simulink model "TestStructure"  (R2023b)
settings: Solver=FixedStepDiscrete  StartTime=0.0  StopTime=inf  FixedStep=SampleTime  RelTol=1e-3
InitFcn:
  | SampleTime = 0.001;
  | ButtonValue=0;
  | load("BusConfig.mat");
undefined symbols (not defined in the file): DiscIntNeverNeededParam
libraries: slrealtimeethercatlib x219, dspfdesign x28, dspstat3 x23, simulink x21, slpidlib x10, dspswit3 x8, commfilt2 x2, dspsigops x1
(part 5 of 8)

== system TestStructure/Robot/MotorPositonInit1/Subsystem3 ==
  MotorDesirePos : Inport
  MotorPos : Inport  Port=2
  MotorVel : Inport  Port=3
  Discrete PID Controller : slpidlib/PID Controller  Controller=PID  Form=Parallel  TimeDomain=Discrete-time  UseExternalTs=off  SampleTime=-1  IntegratorMethod=Forward Euler  FilterMethod=Forward Euler  ControllerParametersSource=internal  P=220  I=1  UseKiTs=off  D=0.5  N=100  UseFilter=on  TunerSelectOption=Transfer Function Based (PID Tuner App)  InitialConditionSource=internal  InitialConditionForIntegrator=0  InitialConditionForFilter=0  DifferentiatorICPrevScaledInput=0  ExternalReset=none  TrackingMode=off  Kt=1  LimitOutput=off  SatLimitsSource=internal  UpperSaturationLimit=inf  LowerSaturationLimit=-inf  LinearizeAsGain=off  AntiWindupMode=none  Kb=1  LimitIntegrator=off  UpperIntegratorSaturationLimit=inf  LowerIntegratorSaturationLimit=-inf  POutMin=[]  POutMax=[]  IOutMin=[]  IOutMax=[]  DOutMin=[]  DOutMax=[]  NOutMin=[]  NOutMax=[]  SumOutMin=[]  SumOutMax=[]  SaturationOutMin=[]  SaturationOutMax=[]  PParamMin=[]  PParamMax=[]  IParamMin=[]  IParamMax=[]  DParamMin=[]  DParamMax=[]  NParamMin=[]  NParamMax=[]  KbParamMin=[]  KbParamMax=[]  KtParamMin=[]  KtParamMax=[]  KbOutMin=[]  KbOutMax=[]  KtOutMin=[]  KtOutMax=[]  IntegratorOutMin=[]  IntegratorOutMax=[]  FilterOutMin=[]  FilterOutMax=[]  SumI1OutMin=[]  SumI1OutMax=[]  SumI2OutMin=[]  SumI2OutMax=[]  SumI3OutMin=[]  SumI3OutMax=[]  SumI4OutMin=[]  SumI4OutMax=[]  SumDOutMin=[]  SumDOutMax=[]  DifferentiatorOutMin=[]  DifferentiatorOutMax=[]  FilterDiffOutCoefMin=[]  FilterDiffOutCoefMax=[]  ReciprocalOutMin=[]  ReciprocalOutMax=[]  SumDenOutMin=[]  SumDenOutMax=[]  SumNumOutMin=[]  SumNumOutMax=[]  DivideOutMin=[]  DivideOutMax=[]  UdiffTsProdOutMin=[]  UdiffTsProdOutMax=[]  NTsProdOutMin=[]  NTsProdOutMax=[]  UintegralTsProdOutMin=[]  UintegralTsProdOutMax=[]  UngainTsProdOutMin=[]  UngainTsProdOutMax=[]  ClampingZeroOutDataTypeStr=Inherit: Inherit via back propagation  ClampingZeroOutMin=[]  ClampingZeroOutMax=[]  FilterDenConstantOutDataTypeStr=Inherit: Inherit via back propagation  FilterDenConstantOutMin=[]  FilterDenConstantOutMax=[]  PCopyOutDataTypeStr=Inherit: Inherit via back propagation  PCopyOutMin=[]  PCopyOutMax=[]  NCopyOutDataTypeStr=Inherit: Inherit via back propagation  NCopyOutMin=[]  NCopyOutMax=[]  IntegratorContinuousStateAttributes=''  IntegratorStateMustResolveToSignalObject=off  IntegratorRTWStateStorageClass=Auto  FilterContinuousStateAttributes=''  FilterStateMustResolveToSignalObject=off  FilterRTWStateStorageClass=Auto  ParallelPVariant=InternalParameters  IdealPVariant=Disabled  IVariant=InternalParameters  DVariant=InternalParameters  IntegratorVariant=Discrete  SatVariant=Disabled  AWVariant=Passthrough  PCopyVariant=Disabled  TRVariant=Disabled  FdbkBlocksVariant=Forward  IdealPFdbkVariant=Disabled  SatFdbkVariant=Disabled  DerivativeFilterVariant=ForwardEulerFilter  NVariant=InternalParameters  NCopyVariant=Disabled  FilterICVariant=InternalICsFilter  IntegratorICVariant=InternalICs  ExternalResetVariant=Disabled  TRSumVariant=Passthrough  SumFdbkVariant=Disabled  SumVariant=Sum_PID  TsampFilterVariant=InternalTs  TsampNgainVariant=Passthrough  TsampIntegralVariant=Disabled_SignalSpec  ExternalSaturationOutDataTypeStr=Inherit: Same as second input
      settings: LibrarySourceBlock=simulink/Discrete/Discrete PID Controller
  Discrete PID Controller1 : slpidlib/PID Controller  Controller=PD  Form=Parallel  TimeDomain=Discrete-time  UseExternalTs=off  SampleTime=-1  IntegratorMethod=Forward Euler  FilterMethod=Forward Euler  ControllerParametersSource=internal  P=0.0035  I=1  UseKiTs=off  D=0.00005  N=100  UseFilter=on  TunerSelectOption=Transfer Function Based (PID Tuner App)  InitialConditionSource=internal  InitialConditionForIntegrator=0  InitialConditionForFilter=0  DifferentiatorICPrevScaledInput=0  ExternalReset=none  TrackingMode=off  Kt=1  LimitOutput=on  SatLimitsSource=internal  UpperSaturationLimit=15  LowerSaturationLimit=-15  LinearizeAsGain=off  AntiWindupMode=none  Kb=1  LimitIntegrator=off  UpperIntegratorSaturationLimit=inf  LowerIntegratorSaturationLimit=-inf  POutMin=[]  POutMax=[]  IOutMin=[]  IOutMax=[]  DOutMin=[]  DOutMax=[]  NOutMin=[]  NOutMax=[]  SumOutMin=[]  SumOutMax=[]  SaturationOutMin=[]  SaturationOutMax=[]  PParamMin=[]  PParamMax=[]  IParamMin=[]  IParamMax=[]  DParamMin=[]  DParamMax=[]  NParamMin=[]  NParamMax=[]  KbParamMin=[]  KbParamMax=[]  KtParamMin=[]  KtParamMax=[]  KbOutMin=[]  KbOutMax=[]  KtOutMin=[]  KtOutMax=[]  IntegratorOutMin=[]  IntegratorOutMax=[]  FilterOutMin=[]  FilterOutMax=[]  SumI1OutMin=[]  SumI1OutMax=[]  SumI2OutMin=[]  SumI2OutMax=[]  SumI3OutMin=[]  SumI3OutMax=[]  SumI4OutMin=[]  SumI4OutMax=[]  SumDOutMin=[]  SumDOutMax=[]  DifferentiatorOutMin=[]  DifferentiatorOutMax=[]  FilterDiffOutCoefMin=[]  FilterDiffOutCoefMax=[]  ReciprocalOutMin=[]  ReciprocalOutMax=[]  SumDenOutMin=[]  SumDenOutMax=[]  SumNumOutMin=[]  SumNumOutMax=[]  DivideOutMin=[]  DivideOutMax=[]  UdiffTsProdOutMin=[]  UdiffTsProdOutMax=[]  NTsProdOutMin=[]  NTsProdOutMax=[]  UintegralTsProdOutMin=[]  UintegralTsProdOutMax=[]  UngainTsProdOutMin=[]  UngainTsProdOutMax=[]  ClampingZeroOutDataTypeStr=Inherit: Inherit via back propagation  ClampingZeroOutMin=[]  ClampingZeroOutMax=[]  FilterDenConstantOutDataTypeStr=Inherit: Inherit via back propagation  FilterDenConstantOutMin=[]  FilterDenConstantOutMax=[]  PCopyOutDataTypeStr=Inherit: Inherit via back propagation  PCopyOutMin=[]  PCopyOutMax=[]  NCopyOutDataTypeStr=Inherit: Inherit via back propagation  NCopyOutMin=[]  NCopyOutMax=[]  IntegratorContinuousStateAttributes=''  IntegratorStateMustResolveToSignalObject=off  IntegratorRTWStateStorageClass=Auto  FilterContinuousStateAttributes=''  FilterStateMustResolveToSignalObject=off  FilterRTWStateStorageClass=Auto  ParallelPVariant=InternalParameters  IdealPVariant=Disabled  IVariant=Disabled  DVariant=InternalParameters  IntegratorVariant=Disabled  SatVariant=Enabled  AWVariant=Disabled  PCopyVariant=Disabled  TRVariant=Disabled  FdbkBlocksVariant=Forward  IdealPFdbkVariant=Disabled  SatFdbkVariant=Disabled  DerivativeFilterVariant=ForwardEulerFilter  NVariant=InternalParameters  NCopyVariant=Disabled  FilterICVariant=InternalICsFilter  IntegratorICVariant=Disabled  ExternalResetVariant=Disabled  TRSumVariant=Passthrough  SumFdbkVariant=Disabled  SumVariant=Sum_PD  TsampFilterVariant=InternalTs  TsampNgainVariant=Passthrough  TsampIntegralVariant=Disabled_SignalSpec  ExternalSaturationOutDataTypeStr=Inherit: Same as second input
      settings: LibrarySourceBlock=simulink/Discrete/Discrete PID Controller
  Saturation1 : Saturate  UpperLimit=60  LowerLimit=-60
  Sum : Sum  Inputs=|+-
  Sum1 : Sum  Inputs=|+-
  MotorTorque : Outport
  wires:
  Discrete PID Controller1/1 -> MotorTorque/1
  Sum/1 -> Discrete PID Controller/1
  Saturation1/1 -> Sum1/2
  Discrete PID Controller/1 -> Sum1/1
  Sum1/1 -> Discrete PID Controller1/1
  MotorDesirePos/1 -> Sum/1
  MotorVel/1 -> Saturation1/1
  MotorPos/1 -> Sum/2

== system TestStructure/Robot/MotorPositonInit1/Subsystem4 ==
  MotorDesirePos : Inport
  MotorPos : Inport  Port=2
  MotorVel : Inport  Port=3
  Discrete PID Controller : slpidlib/PID Controller  Controller=PID  Form=Parallel  TimeDomain=Discrete-time  UseExternalTs=off  SampleTime=-1  IntegratorMethod=Forward Euler  FilterMethod=Forward Euler  ControllerParametersSource=internal  P=220  I=1  UseKiTs=off  D=2  N=100  UseFilter=on  TunerSelectOption=Transfer Function Based (PID Tuner App)  InitialConditionSource=internal  InitialConditionForIntegrator=0  InitialConditionForFilter=0  DifferentiatorICPrevScaledInput=0  ExternalReset=none  TrackingMode=off  Kt=1  LimitOutput=off  SatLimitsSource=internal  UpperSaturationLimit=inf  LowerSaturationLimit=-inf  LinearizeAsGain=off  AntiWindupMode=none  Kb=1  LimitIntegrator=off  UpperIntegratorSaturationLimit=inf  LowerIntegratorSaturationLimit=-inf  POutMin=[]  POutMax=[]  IOutMin=[]  IOutMax=[]  DOutMin=[]  DOutMax=[]  NOutMin=[]  NOutMax=[]  SumOutMin=[]  SumOutMax=[]  SaturationOutMin=[]  SaturationOutMax=[]  PParamMin=[]  PParamMax=[]  IParamMin=[]  IParamMax=[]  DParamMin=[]  DParamMax=[]  NParamMin=[]  NParamMax=[]  KbParamMin=[]  KbParamMax=[]  KtParamMin=[]  KtParamMax=[]  KbOutMin=[]  KbOutMax=[]  KtOutMin=[]  KtOutMax=[]  IntegratorOutMin=[]  IntegratorOutMax=[]  FilterOutMin=[]  FilterOutMax=[]  SumI1OutMin=[]  SumI1OutMax=[]  SumI2OutMin=[]  SumI2OutMax=[]  SumI3OutMin=[]  SumI3OutMax=[]  SumI4OutMin=[]  SumI4OutMax=[]  SumDOutMin=[]  SumDOutMax=[]  DifferentiatorOutMin=[]  DifferentiatorOutMax=[]  FilterDiffOutCoefMin=[]  FilterDiffOutCoefMax=[]  ReciprocalOutMin=[]  ReciprocalOutMax=[]  SumDenOutMin=[]  SumDenOutMax=[]  SumNumOutMin=[]  SumNumOutMax=[]  DivideOutMin=[]  DivideOutMax=[]  UdiffTsProdOutMin=[]  UdiffTsProdOutMax=[]  NTsProdOutMin=[]  NTsProdOutMax=[]  UintegralTsProdOutMin=[]  UintegralTsProdOutMax=[]  UngainTsProdOutMin=[]  UngainTsProdOutMax=[]  ClampingZeroOutDataTypeStr=Inherit: Inherit via back propagation  ClampingZeroOutMin=[]  ClampingZeroOutMax=[]  FilterDenConstantOutDataTypeStr=Inherit: Inherit via back propagation  FilterDenConstantOutMin=[]  FilterDenConstantOutMax=[]  PCopyOutDataTypeStr=Inherit: Inherit via back propagation  PCopyOutMin=[]  PCopyOutMax=[]  NCopyOutDataTypeStr=Inherit: Inherit via back propagation  NCopyOutMin=[]  NCopyOutMax=[]  IntegratorContinuousStateAttributes=''  IntegratorStateMustResolveToSignalObject=off  IntegratorRTWStateStorageClass=Auto  FilterContinuousStateAttributes=''  FilterStateMustResolveToSignalObject=off  FilterRTWStateStorageClass=Auto  ParallelPVariant=InternalParameters  IdealPVariant=Disabled  IVariant=InternalParameters  DVariant=InternalParameters  IntegratorVariant=Discrete  SatVariant=Disabled  AWVariant=Passthrough  PCopyVariant=Disabled  TRVariant=Disabled  FdbkBlocksVariant=Forward  IdealPFdbkVariant=Disabled  SatFdbkVariant=Disabled  DerivativeFilterVariant=ForwardEulerFilter  NVariant=InternalParameters  NCopyVariant=Disabled  FilterICVariant=InternalICsFilter  IntegratorICVariant=InternalICs  ExternalResetVariant=Disabled  TRSumVariant=Passthrough  SumFdbkVariant=Disabled  SumVariant=Sum_PID  TsampFilterVariant=InternalTs  TsampNgainVariant=Passthrough  TsampIntegralVariant=Disabled_SignalSpec  ExternalSaturationOutDataTypeStr=Inherit: Same as second input
      settings: LibrarySourceBlock=simulink/Discrete/Discrete PID Controller
  Discrete PID Controller1 : slpidlib/PID Controller  Controller=PD  Form=Parallel  TimeDomain=Discrete-time  UseExternalTs=off  SampleTime=-1  IntegratorMethod=Forward Euler  FilterMethod=Forward Euler  ControllerParametersSource=internal  P=0.0035  I=1  UseKiTs=off  D=0.00005  N=100  UseFilter=on  TunerSelectOption=Transfer Function Based (PID Tuner App)  InitialConditionSource=internal  InitialConditionForIntegrator=0  InitialConditionForFilter=0  DifferentiatorICPrevScaledInput=0  ExternalReset=none  TrackingMode=off  Kt=1  LimitOutput=on  SatLimitsSource=internal  UpperSaturationLimit=15  LowerSaturationLimit=-15  LinearizeAsGain=off  AntiWindupMode=none  Kb=1  LimitIntegrator=off  UpperIntegratorSaturationLimit=inf  LowerIntegratorSaturationLimit=-inf  POutMin=[]  POutMax=[]  IOutMin=[]  IOutMax=[]  DOutMin=[]  DOutMax=[]  NOutMin=[]  NOutMax=[]  SumOutMin=[]  SumOutMax=[]  SaturationOutMin=[]  SaturationOutMax=[]  PParamMin=[]  PParamMax=[]  IParamMin=[]  IParamMax=[]  DParamMin=[]  DParamMax=[]  NParamMin=[]  NParamMax=[]  KbParamMin=[]  KbParamMax=[]  KtParamMin=[]  KtParamMax=[]  KbOutMin=[]  KbOutMax=[]  KtOutMin=[]  KtOutMax=[]  IntegratorOutMin=[]  IntegratorOutMax=[]  FilterOutMin=[]  FilterOutMax=[]  SumI1OutMin=[]  SumI1OutMax=[]  SumI2OutMin=[]  SumI2OutMax=[]  SumI3OutMin=[]  SumI3OutMax=[]  SumI4OutMin=[]  SumI4OutMax=[]  SumDOutMin=[]  SumDOutMax=[]  DifferentiatorOutMin=[]  DifferentiatorOutMax=[]  FilterDiffOutCoefMin=[]  FilterDiffOutCoefMax=[]  ReciprocalOutMin=[]  ReciprocalOutMax=[]  SumDenOutMin=[]  SumDenOutMax=[]  SumNumOutMin=[]  SumNumOutMax=[]  DivideOutMin=[]  DivideOutMax=[]  UdiffTsProdOutMin=[]  UdiffTsProdOutMax=[]  NTsProdOutMin=[]  NTsProdOutMax=[]  UintegralTsProdOutMin=[]  UintegralTsProdOutMax=[]  UngainTsProdOutMin=[]  UngainTsProdOutMax=[]  ClampingZeroOutDataTypeStr=Inherit: Inherit via back propagation  ClampingZeroOutMin=[]  ClampingZeroOutMax=[]  FilterDenConstantOutDataTypeStr=Inherit: Inherit via back propagation  FilterDenConstantOutMin=[]  FilterDenConstantOutMax=[]  PCopyOutDataTypeStr=Inherit: Inherit via back propagation  PCopyOutMin=[]  PCopyOutMax=[]  NCopyOutDataTypeStr=Inherit: Inherit via back propagation  NCopyOutMin=[]  NCopyOutMax=[]  IntegratorContinuousStateAttributes=''  IntegratorStateMustResolveToSignalObject=off  IntegratorRTWStateStorageClass=Auto  FilterContinuousStateAttributes=''  FilterStateMustResolveToSignalObject=off  FilterRTWStateStorageClass=Auto  ParallelPVariant=InternalParameters  IdealPVariant=Disabled  IVariant=Disabled  DVariant=InternalParameters  IntegratorVariant=Disabled  SatVariant=Enabled  AWVariant=Disabled  PCopyVariant=Disabled  TRVariant=Disabled  FdbkBlocksVariant=Forward  IdealPFdbkVariant=Disabled  SatFdbkVariant=Disabled  DerivativeFilterVariant=ForwardEulerFilter  NVariant=InternalParameters  NCopyVariant=Disabled  FilterICVariant=InternalICsFilter  IntegratorICVariant=Disabled  ExternalResetVariant=Disabled  TRSumVariant=Passthrough  SumFdbkVariant=Disabled  SumVariant=Sum_PD  TsampFilterVariant=InternalTs  TsampNgainVariant=Passthrough  TsampIntegralVariant=Disabled_SignalSpec  ExternalSaturationOutDataTypeStr=Inherit: Same as second input
      settings: LibrarySourceBlock=simulink/Discrete/Discrete PID Controller
  Saturation1 : Saturate  UpperLimit=60  LowerLimit=-60
  Sum : Sum  Inputs=|+-
  Sum1 : Sum  Inputs=|+-
  MotorTorque : Outport
  wires:
  Discrete PID Controller1/1 -> MotorTorque/1
  Sum/1 -> Discrete PID Controller/1
  Saturation1/1 -> Sum1/2
  Discrete PID Controller/1 -> Sum1/1
  Sum1/1 -> Discrete PID Controller1/1
  MotorDesirePos/1 -> Sum/1
  MotorVel/1 -> Saturation1/1
  MotorPos/1 -> Sum/2

== system TestStructure/Bus/Subsystem6/Enabled Subsystem/Subsystem ==
  In1 : Inport
  In2 : Inport  Port=2
  In3 : Inport  Port=3
  In4 : Inport  Port=4
  EtherCAT PDO Receive1 : slrealtimeethercatlib/EtherCAT PDO Receive  Priority=2  sig_name=Box 1 (PIC32 EtherCAT Slave01).INPUTS process data mapping.FORCE1  sig_offset=696  sig_type=single  type_size=32  sig_dim=1  device_id=0  sample_time=0.001
  EtherCAT PDO Receive2 : slrealtimeethercatlib/EtherCAT PDO Receive  Priority=2  sig_name=Box 1 (PIC32 EtherCAT Slave01).INPUTS process data mapping.FORCE2  sig_offset=728  sig_type=single  type_size=32  sig_dim=1  device_id=0  sample_time=0.001000
  EtherCAT PDO Receive3 : slrealtimeethercatlib/EtherCAT PDO Receive  Priority=2  sig_name=Box 1 (PIC32 EtherCAT Slave01).INPUTS process data mapping.IMU1_X  sig_offset=952  sig_type=single  type_size=32  sig_dim=1  device_id=0  sample_time=0.001000
  EtherCAT PDO Receive4 : slrealtimeethercatlib/EtherCAT PDO Receive  Priority=2  sig_name=Box 1 (PIC32 EtherCAT Slave01).INPUTS process data mapping.IMU1_Y  sig_offset=984  sig_type=single  type_size=32  sig_dim=1  device_id=0  sample_time=0.001000
  EtherCAT PDO Receive5 : slrealtimeethercatlib/EtherCAT PDO Receive  Priority=2  sig_name=Box 1 (PIC32 EtherCAT Slave01).INPUTS process data mapping.IMU1_Z  sig_offset=1016  sig_type=single  type_size=32  sig_dim=1  device_id=0  sample_time=0.001000
  EtherCAT PDO Receive6 : slrealtimeethercatlib/EtherCAT PDO Receive  Priority=2  sig_name=Box 1 (PIC32 EtherCAT Slave01).INPUTS process data mapping.IMU2_X  sig_offset=1048  sig_type=single  type_size=32  sig_dim=1  device_id=0  sample_time=0.001000
  EtherCAT PDO Receive7 : slrealtimeethercatlib/EtherCAT PDO Receive  Priority=2  sig_name=Box 1 (PIC32 EtherCAT Slave01).INPUTS process data mapping.FORCE3  sig_offset=760  sig_type=single  type_size=32  sig_dim=1  device_id=0  sample_time=0.001000
  EtherCAT PDO Receive8 : slrealtimeethercatlib/EtherCAT PDO Receive  Priority=2  sig_name=Box 1 (PIC32 EtherCAT Slave01).INPUTS process data mapping.FORCE3  sig_offset=760  sig_type=single  type_size=32  sig_dim=1  device_id=0  sample_time=0.001000
  EtherCAT PDO Receive9 : slrealtimeethercatlib/EtherCAT PDO Receive  Priority=2  sig_name=Box 1 (PIC32 EtherCAT Slave01).INPUTS process data mapping.FORCE3  sig_offset=760  sig_type=single  type_size=32  sig_dim=1  device_id=0  sample_time=0.001000
  EtherCAT PDO Transmit{,1..3} (4 alike) : slrealtimeethercatlib/EtherCAT PDO Transmit  Priority=5  sig_name=Drive 2 (Elmo Drive ).Outputs.Target Torque  sig_offset=12496  sig_type=int16  type_size=16  sig_dim=1  device_id=0  sample_time=0.001000
  Out1 : Outport
  Out2 : Outport  Port=2
  Out3 : Outport  Port=3
  Out4 : Outport  Port=4
  Out5 : Outport  Port=5
  Out6 : Outport  Port=6
  Out7 : Outport  Port=7
  Out8 : Outport  Port=8
  Out9 : Outport  Port=9
  wires:
  EtherCAT PDO Receive1/1 -> Out1/1
  EtherCAT PDO Receive2/1 -> Out2/1
  EtherCAT PDO Receive3/1 -> Out3/1
  EtherCAT PDO Receive4/1 -> Out4/1
  EtherCAT PDO Receive5/1 -> Out5/1
  EtherCAT PDO Receive6/1 -> Out6/1
  EtherCAT PDO Receive7/1 -> Out7/1
  EtherCAT PDO Receive8/1 -> Out8/1
  EtherCAT PDO Receive9/1 -> Out9/1
  In1/1 -> EtherCAT PDO Transmit/1
  In2/1 -> EtherCAT PDO Transmit1/1
  In4/1 -> EtherCAT PDO Transmit2/1
  In3/1 -> EtherCAT PDO Transmit3/1

== system TestStructure/Bus/Subsystem6/Enabled Subsystem/Subsystem1 ==
  In1 : Inport
  EtherCAT PDO Receive1 : slrealtimeethercatlib/EtherCAT PDO Receive  Priority=2  Commented=on  sig_name=Drive 2 (Elmo Drive ).Inputs.Position actual value  sig_offset=12496  sig_type=int32  type_size=32  sig_dim=1  device_id=0  sample_time=0.001000
  EtherCAT PDO Receive2 : slrealtimeethercatlib/EtherCAT PDO Receive  Priority=2  Commented=on  sig_name=Drive 2 (Elmo Drive ).Inputs_1.Velocity actual value  sig_offset=12576  sig_type=int32  type_size=32  sig_dim=1  device_id=0  sample_time=0.001000
  EtherCAT PDO Receive3 : slrealtimeethercatlib/EtherCAT PDO Receive  Priority=2  Commented=on  sig_name=Drive 2 (Elmo Drive ).Inputs.Torque actual value  sig_offset=12528  sig_type=int16  type_size=16  sig_dim=1  device_id=0  sample_time=0.001000
  EtherCAT PDO Receive4 : slrealtimeethercatlib/EtherCAT PDO Receive  Priority=2  Commented=on  sig_name=Drive 2 (Elmo Drive ).Inputs_2.DC link circuit voltage  sig_offset=12608  sig_type=uint32  type_size=32  sig_dim=1  device_id=0  sample_time=0.001000
  EtherCAT PDO Receive5 : slrealtimeethercatlib/EtherCAT PDO Receive  Priority=2  Commented=on  sig_name=Drive 2 (Elmo Drive ).Inputs.Mode of operation display  sig_offset=12560  sig_type=int8  type_size=8  sig_dim=1  device_id=0  sample_time=0.001000
  EtherCAT PDO Transmit : slrealtimeethercatlib/EtherCAT PDO Transmit  Priority=5  sig_name=Drive 3 (Elmo Drive ).Outputs.Target Torque  sig_offset=1432  sig_type=int16  type_size=16  sig_dim=1  device_id=0  sample_time=0.001000
  Out1 : Outport
  Out2 : Outport  Port=2
  Out3 : Outport  Port=3
  Out4 : Outport  Port=4
  Out5 : Outport  Port=5
  wires:
  In1/1 -> EtherCAT PDO Transmit/1
  EtherCAT PDO Receive5/1 -> Out5/1
  EtherCAT PDO Receive4/1 -> Out4/1
  EtherCAT PDO Receive3/1 -> Out3/1
  EtherCAT PDO Receive2/1 -> Out2/1
  EtherCAT PDO Receive1/1 -> Out1/1

== system TestStructure/Bus/Subsystem6/Enabled Subsystem/Subsystem10 ==
  EtherCAT PDO Receive1 : slrealtimeethercatlib/EtherCAT PDO Receive  Priority=2  sig_name=Box 1 (PIC32 EtherCAT Slave01).INPUTS process data mapping.FORCE1  sig_offset=696  sig_type=single  type_size=32  sig_dim=1  device_id=0  sample_time=0.001000
  EtherCAT PDO Receive2 : slrealtimeethercatlib/EtherCAT PDO Receive  Priority=2  sig_name=Box 1 (PIC32 EtherCAT Slave01).INPUTS process data mapping.FORCE2  sig_offset=728  sig_type=single  type_size=32  sig_dim=1  device_id=0  sample_time=0.001000
  EtherCAT PDO Receive3 : slrealtimeethercatlib/EtherCAT PDO Receive  Priority=2  sig_name=Box 1 (PIC32 EtherCAT Slave01).INPUTS process data mapping.IMU1_X  sig_offset=952  sig_type=single  type_size=32  sig_dim=1  device_id=0  sample_time=0.001000
  EtherCAT PDO Receive4 : slrealtimeethercatlib/EtherCAT PDO Receive  Priority=2  sig_name=Box 1 (PIC32 EtherCAT Slave01).INPUTS process data mapping.IMU1_Y  sig_offset=984  sig_type=single  type_size=32  sig_dim=1  device_id=0  sample_time=0.001000
  EtherCAT PDO Receive5 : slrealtimeethercatlib/EtherCAT PDO Receive  Priority=2  sig_name=Box 1 (PIC32 EtherCAT Slave01).INPUTS process data mapping.IMU1_Z  sig_offset=1016  sig_type=single  type_size=32  sig_dim=1  device_id=0  sample_time=0.001000
  EtherCAT PDO Receive6 : slrealtimeethercatlib/EtherCAT PDO Receive  Priority=2  sig_name=Box 1 (PIC32 EtherCAT Slave01).INPUTS process data mapping.IMU2_X  sig_offset=1048  sig_type=single  type_size=32  sig_dim=1  device_id=0  sample_time=0.001000
  EtherCAT PDO Receive7 : slrealtimeethercatlib/EtherCAT PDO Receive  Priority=2  sig_name=Box 1 (PIC32 EtherCAT Slave01).INPUTS process data mapping.FORCE3  sig_offset=760  sig_type=single  type_size=32  sig_dim=1  device_id=0  sample_time=0.001000
  Out1 : Outport
  Out2 : Outport  Port=2
  Out3 : Outport  Port=3
  Out4 : Outport  Port=4
  Out5 : Outport  Port=5
  Out6 : Outport  Port=6
  Out7 : Outport  Port=7
  wires:
  EtherCAT PDO Receive1/1 -> Out1/1
  EtherCAT PDO Receive2/1 -> Out2/1
  EtherCAT PDO Receive3/1 -> Out3/1
  EtherCAT PDO Receive4/1 -> Out4/1
  EtherCAT PDO Receive5/1 -> Out5/1
  EtherCAT PDO Receive6/1 -> Out6/1
  EtherCAT PDO Receive7/1 -> Out7/1

== system TestStructure/Bus/Subsystem6/Enabled Subsystem/Subsystem11 ==
  EtherCAT PDO Receive1 : slrealtimeethercatlib/EtherCAT PDO Receive  Priority=2  sig_name=Box 1 (PIC32 EtherCAT Slave01).INPUTS process data mapping.FORCE1  sig_offset=696  sig_type=single  type_size=32  sig_dim=1  device_id=0  sample_time=0.001000
  EtherCAT PDO Receive2 : slrealtimeethercatlib/EtherCAT PDO Receive  Priority=2  sig_name=Box 1 (PIC32 EtherCAT Slave01).INPUTS process data mapping.FORCE2  sig_offset=728  sig_type=single  type_size=32  sig_dim=1  device_id=0  sample_time=0.001000
  EtherCAT PDO Receive3 : slrealtimeethercatlib/EtherCAT PDO Receive  Priority=2  sig_name=Box 1 (PIC32 EtherCAT Slave01).INPUTS process data mapping.IMU1_X  sig_offset=952  sig_type=single  type_size=32  sig_dim=1  device_id=0  sample_time=0.001000
  EtherCAT PDO Receive4 : slrealtimeethercatlib/EtherCAT PDO Receive  Priority=2  sig_name=Box 1 (PIC32 EtherCAT Slave01).INPUTS process data mapping.IMU1_Y  sig_offset=984  sig_type=single  type_size=32  sig_dim=1  device_id=0  sample_time=0.001000
  EtherCAT PDO Receive5 : slrealtimeethercatlib/EtherCAT PDO Receive  Priority=2  sig_name=Box 1 (PIC32 EtherCAT Slave01).INPUTS process data mapping.IMU1_Z  sig_offset=1016  sig_type=single  type_size=32  sig_dim=1  device_id=0  sample_time=0.001000
  EtherCAT PDO Receive6 : slrealtimeethercatlib/EtherCAT PDO Receive  Priority=2  sig_name=Box 1 (PIC32 EtherCAT Slave01).INPUTS process data mapping.IMU2_X  sig_offset=1048  sig_type=single  type_size=32  sig_dim=1  device_id=0  sample_time=0.001000
  EtherCAT PDO Receive7 : slrealtimeethercatlib/EtherCAT PDO Receive  Priority=2  sig_name=Box 1 (PIC32 EtherCAT Slave01).INPUTS process data mapping.FORCE3  sig_offset=760  sig_type=single  type_size=32  sig_dim=1  device_id=0  sample_time=0.001000
  Out1 : Outport
  Out2 : Outport  Port=2
  Out3 : Outport  Port=3
  Out4 : Outport  Port=4
  Out5 : Outport  Port=5
  Out6 : Outport  Port=6
  Out7 : Outport  Port=7
  wires:
  EtherCAT PDO Receive1/1 -> Out1/1
  EtherCAT PDO Receive2/1 -> Out2/1
  EtherCAT PDO Receive3/1 -> Out3/1
  EtherCAT PDO Receive4/1 -> Out4/1
  EtherCAT PDO Receive5/1 -> Out5/1
  EtherCAT PDO Receive6/1 -> Out6/1
  EtherCAT PDO Receive7/1 -> Out7/1

== system TestStructure/Bus/Subsystem6/Enabled Subsystem/Subsystem2 ==
  In1 : Inport
  EtherCAT PDO Receive1 : slrealtimeethercatlib/EtherCAT PDO Receive  Priority=2  Commented=on  sig_name=Drive 4 (Elmo Drive ).Inputs.Position actual value  sig_offset=37072  sig_type=int32  type_size=32  sig_dim=1  device_id=0  sample_time=0.001000
  EtherCAT PDO Receive2 : slrealtimeethercatlib/EtherCAT PDO Receive  Priority=2  Commented=on  sig_name=Drive 4 (Elmo Drive ).Inputs_1.Velocity actual value  sig_offset=37152  sig_type=int32  type_size=32  sig_dim=1  device_id=0  sample_time=0.001000
  EtherCAT PDO Receive3 : slrealtimeethercatlib/EtherCAT PDO Receive  Priority=2  Commented=on  sig_name=Drive 4 (Elmo Drive ).Inputs.Torque actual value  sig_offset=37104  sig_type=int16  type_size=16  sig_dim=1  device_id=0  sample_time=0.001000
  EtherCAT PDO Receive4 : slrealtimeethercatlib/EtherCAT PDO Receive  Priority=2  Commented=on  sig_name=Drive 4 (Elmo Drive ).Inputs_2.DC link circuit voltage  sig_offset=37184  sig_type=uint32  type_size=32  sig_dim=1  device_id=0  sample_time=0.001000
  EtherCAT PDO Receive5 : slrealtimeethercatlib/EtherCAT PDO Receive  Priority=2  Commented=on  sig_name=Drive 4 (Elmo Drive ).Inputs.Mode of operation display  sig_offset=37136  sig_type=int8  type_size=8  sig_dim=1  device_id=0  sample_time=0.001000
  EtherCAT PDO Transmit : slrealtimeethercatlib/EtherCAT PDO Transmit  Priority=5  sig_name=Drive 6 (Elmo Drive ).Outputs.Target Torque  sig_offset=13232  sig_type=int16  type_size=16  sig_dim=1  device_id=0  sample_time=0.001000
  Out1 : Outport
  Out2 : Outport  Port=2
  Out3 : Outport  Port=3
  Out4 : Outport  Port=4
  Out5 : Outport  Port=5
  wires:
  In1/1 -> EtherCAT PDO Transmit/1
  EtherCAT PDO Receive5/1 -> Out5/1
  EtherCAT PDO Receive4/1 -> Out4/1
  EtherCAT PDO Receive3/1 -> Out3/1
  EtherCAT PDO Receive2/1 -> Out2/1
  EtherCAT PDO Receive1/1 -> Out1/1

== system TestStructure/Bus/Subsystem6/Enabled Subsystem/Subsystem3 ==
  In1 : Inport
  EtherCAT PDO Receive1 : slrealtimeethercatlib/EtherCAT PDO Receive  Priority=2  sig_name=Drive 2 (Elmo Drive ).Inputs.Position actual value  sig_offset=12496  sig_type=int32  type_size=32  sig_dim=1  device_id=0  sample_time=0.001000
  EtherCAT PDO Receive2 : slrealtimeethercatlib/EtherCAT PDO Receive  Priority=2  sig_name=Drive 2 (Elmo Drive ).Inputs_1.Velocity actual value  sig_offset=12576  sig_type=int32  type_size=32  sig_dim=1  device_id=0  sample_time=0.001000
  EtherCAT PDO Receive3 : slrealtimeethercatlib/EtherCAT PDO Receive  Priority=2  sig_name=Drive 2 (Elmo Drive ).Inputs.Torque actual value  sig_offset=12528  sig_type=int16  type_size=16  sig_dim=1  device_id=0  sample_time=0.001000
  EtherCAT PDO Receive4 : slrealtimeethercatlib/EtherCAT PDO Receive  Priority=2  sig_name=Drive 2 (Elmo Drive ).Inputs_2.DC link circuit voltage  sig_offset=12608  sig_type=uint32  type_size=32  sig_dim=1  device_id=0  sample_time=0.001000
  EtherCAT PDO Receive5 : slrealtimeethercatlib/EtherCAT PDO Receive  Priority=2  sig_name=Drive 2 (Elmo Drive ).Inputs.Mode of operation display  sig_offset=12560  sig_type=int8  type_size=8  sig_dim=1  device_id=0  sample_time=0.001000
  EtherCAT PDO Transmit : slrealtimeethercatlib/EtherCAT PDO Transmit  Priority=5  sig_name=Drive 2 (Elmo Drive ).Outputs.Target Torque  sig_offset=12496  sig_type=int16  type_size=16  sig_dim=1  device_id=0  sample_time=0.001000
  Out1 : Outport
  Out2 : Outport  Port=2
  Out3 : Outport  Port=3
  Out4 : Outport  Port=4
  Out5 : Outport  Port=5
  wires:
  In1/1 -> EtherCAT PDO Transmit/1
  EtherCAT PDO Receive5/1 -> Out5/1
  EtherCAT PDO Receive4/1 -> Out4/1
  EtherCAT PDO Receive3/1 -> Out3/1
  EtherCAT PDO Receive2/1 -> Out2/1
  EtherCAT PDO Receive1/1 -> Out1/1

== system TestStructure/Bus/Subsystem6/Enabled Subsystem/Subsystem4 ==
  In1 : Inport
  EtherCAT PDO Receive1 : slrealtimeethercatlib/EtherCAT PDO Receive  Priority=2  sig_name=Drive 2 (Elmo Drive ).Inputs.Position actual value  sig_offset=12496  sig_type=int32  type_size=32  sig_dim=1  device_id=0  sample_time=0.001000
  EtherCAT PDO Receive2 : slrealtimeethercatlib/EtherCAT PDO Receive  Priority=2  sig_name=Drive 2 (Elmo Drive ).Inputs_1.Velocity actual value  sig_offset=12576  sig_type=int32  type_size=32  sig_dim=1  device_id=0  sample_time=0.001000
  EtherCAT PDO Receive3 : slrealtimeethercatlib/EtherCAT PDO Receive  Priority=2  sig_name=Drive 2 (Elmo Drive ).Inputs.Torque actual value  sig_offset=12528  sig_type=int16  type_size=16  sig_dim=1  device_id=0  sample_time=0.001000
  EtherCAT PDO Receive4 : slrealtimeethercatlib/EtherCAT PDO Receive  Priority=2  sig_name=Drive 2 (Elmo Drive ).Inputs_2.DC link circuit voltage  sig_offset=12608  sig_type=uint32  type_size=32  sig_dim=1  device_id=0  sample_time=0.001000
  EtherCAT PDO Receive5 : slrealtimeethercatlib/EtherCAT PDO Receive  Priority=2  sig_name=Drive 2 (Elmo Drive ).Inputs.Mode of operation display  sig_offset=12560  sig_type=int8  type_size=8  sig_dim=1  device_id=0  sample_time=0.001000
  EtherCAT PDO Transmit : slrealtimeethercatlib/EtherCAT PDO Transmit  Priority=5  sig_name=Drive 2 (Elmo Drive ).Outputs.Target Torque  sig_offset=12496  sig_type=int16  type_size=16  sig_dim=1  device_id=0  sample_time=0.001000
  Out1 : Outport
  Out2 : Outport  Port=2
  Out3 : Outport  Port=3
  Out4 : Outport  Port=4
  Out5 : Outport  Port=5
  wires:
  In1/1 -> EtherCAT PDO Transmit/1
  EtherCAT PDO Receive5/1 -> Out5/1
  EtherCAT PDO Receive4/1 -> Out4/1
  EtherCAT PDO Receive3/1 -> Out3/1
  EtherCAT PDO Receive2/1 -> Out2/1
  EtherCAT PDO Receive1/1 -> Out1/1

== system TestStructure/Bus/Subsystem6/Enabled Subsystem/Subsystem5 ==
  EtherCAT PDO Receive1 : slrealtimeethercatlib/EtherCAT PDO Receive  Priority=2  Commented=on  sig_name=Box 1 (PIC32 EtherCAT Slave01).INPUTS process data mapping.FORCE1  sig_offset=696  sig_type=single  type_size=32  sig_dim=1  device_id=0  sample_time=0.001000
  EtherCAT PDO Receive2 : slrealtimeethercatlib/EtherCAT PDO Receive  Priority=2  Commented=on  sig_name=Box 1 (PIC32 EtherCAT Slave01).INPUTS process data mapping.FORCE2  sig_offset=728  sig_type=single  type_size=32  sig_dim=1  device_id=0  sample_time=0.001000
  EtherCAT PDO Receive3 : slrealtimeethercatlib/EtherCAT PDO Receive  Priority=2  Commented=on  sig_name=Box 1 (PIC32 EtherCAT Slave01).INPUTS process data mapping.IMU1_X  sig_offset=952  sig_type=single  type_size=32  sig_dim=1  device_id=0  sample_time=0.001000
  EtherCAT PDO Receive4 : slrealtimeethercatlib/EtherCAT PDO Receive  Priority=2  Commented=on  sig_name=Box 1 (PIC32 EtherCAT Slave01).INPUTS process data mapping.IMU1_Y  sig_offset=984  sig_type=single  type_size=32  sig_dim=1  device_id=0  sample_time=0.001000
  EtherCAT PDO Receive5 : slrealtimeethercatlib/EtherCAT PDO Receive  Priority=2  Commented=on  sig_name=Box 1 (PIC32 EtherCAT Slave01).INPUTS process data mapping.IMU1_Z  sig_offset=1016  sig_type=single  type_size=32  sig_dim=1  device_id=0  sample_time=0.001000
  EtherCAT PDO Receive6 : slrealtimeethercatlib/EtherCAT PDO Receive  Priority=2  Commented=on  sig_name=Box 1 (PIC32 EtherCAT Slave01).INPUTS process data mapping.IMU2_X  sig_offset=1048  sig_type=single  type_size=32  sig_dim=1  device_id=0  sample_time=0.001000
  EtherCAT PDO Receive7 : slrealtimeethercatlib/EtherCAT PDO Receive  Priority=2  Commented=on  sig_name=Box 1 (PIC32 EtherCAT Slave01).INPUTS process data mapping.FORCE3  sig_offset=760  sig_type=single  type_size=32  sig_dim=1  device_id=0  sample_time=0.001000
  Out1 : Outport
  Out2 : Outport  Port=2
  Out3 : Outport  Port=3
  Out4 : Outport  Port=4
  Out5 : Outport  Port=5
  Out6 : Outport  Port=6
  Out7 : Outport  Port=7
  wires:
  EtherCAT PDO Receive1/1 -> Out1/1
  EtherCAT PDO Receive2/1 -> Out2/1
  EtherCAT PDO Receive3/1 -> Out3/1
  EtherCAT PDO Receive4/1 -> Out4/1
  EtherCAT PDO Receive5/1 -> Out5/1
  EtherCAT PDO Receive6/1 -> Out6/1
  EtherCAT PDO Receive7/1 -> Out7/1

== system TestStructure/Bus/Subsystem6/Enabled Subsystem/Subsystem6 ==
  EtherCAT PDO Receive1 : slrealtimeethercatlib/EtherCAT PDO Receive  Priority=2  Commented=on  sig_name=Box 3 (PIC32 EtherCAT Slave01).INPUTS process data mapping.FORCE1  sig_offset=24784  sig_type=single  type_size=32  sig_dim=1  device_id=0  sample_time=0.001000
  EtherCAT PDO Receive2 : slrealtimeethercatlib/EtherCAT PDO Receive  Priority=2  Commented=on  sig_name=Box 3 (PIC32 EtherCAT Slave01).INPUTS process data mapping.FORCE2  sig_offset=24816  sig_type=single  type_size=32  sig_dim=1  device_id=0  sample_time=0.001000
  EtherCAT PDO Receive3 : slrealtimeethercatlib/EtherCAT PDO Receive  Priority=2  Commented=on  sig_name=Box 3 (PIC32 EtherCAT Slave01).INPUTS process data mapping.IMU1_X  sig_offset=25040  sig_type=single  type_size=32  sig_dim=1  device_id=0  sample_time=0.001000
  EtherCAT PDO Receive4 : slrealtimeethercatlib/EtherCAT PDO Receive  Priority=2  Commented=on  sig_name=Box 3 (PIC32 EtherCAT Slave01).INPUTS process data mapping.IMU1_Y  sig_offset=25072  sig_type=single  type_size=32  sig_dim=1  device_id=0  sample_time=0.001000
  EtherCAT PDO Receive5 : slrealtimeethercatlib/EtherCAT PDO Receive  Priority=2  Commented=on  sig_name=Box 3 (PIC32 EtherCAT Slave01).INPUTS process data mapping.IMU1_Z  sig_offset=25104  sig_type=single  type_size=32  sig_dim=1  device_id=0  sample_time=0.001000
  EtherCAT PDO Receive6 : slrealtimeethercatlib/EtherCAT PDO Receive  Priority=2  Commented=on  sig_name=Box 3 (PIC32 EtherCAT Slave01).INPUTS process data mapping.IMU2_X  sig_offset=25136  sig_type=single  type_size=32  sig_dim=1  device_id=0  sample_time=0.001000
  EtherCAT PDO Receive7 : slrealtimeethercatlib/EtherCAT PDO Receive  Priority=2  Commented=on  sig_name=Box 3 (PIC32 EtherCAT Slave01).INPUTS process data mapping.FORCE3  sig_offset=24848  sig_type=single  type_size=32  sig_dim=1  device_id=0  sample_time=0.001000
  Out1 : Outport
  Out2 : Outport  Port=2
  Out3 : Outport  Port=3
  Out4 : Outport  Port=4
  Out5 : Outport  Port=5
  Out6 : Outport  Port=6
  Out7 : Outport  Port=7
  wires:
  EtherCAT PDO Receive1/1 -> Out1/1
  EtherCAT PDO Receive2/1 -> Out2/1
  EtherCAT PDO Receive3/1 -> Out3/1
  EtherCAT PDO Receive4/1 -> Out4/1
  EtherCAT PDO Receive5/1 -> Out5/1
  EtherCAT PDO Receive6/1 -> Out6/1
  EtherCAT PDO Receive7/1 -> Out7/1

== system TestStructure/Bus/Subsystem6/Enabled Subsystem/Subsystem7 ==
  EtherCAT PDO Receive1 : slrealtimeethercatlib/EtherCAT PDO Receive  Priority=2  sig_name=Box 1 (PIC32 EtherCAT Slave01).INPUTS process data mapping.FORCE1  sig_offset=696  sig_type=single  type_size=32  sig_dim=1  device_id=0  sample_time=0.001000
  EtherCAT PDO Receive2 : slrealtimeethercatlib/EtherCAT PDO Receive  Priority=2  sig_name=Box 1 (PIC32 EtherCAT Slave01).INPUTS process data mapping.FORCE2  sig_offset=728  sig_type=single  type_size=32  sig_dim=1  device_id=0  sample_time=0.001000
  EtherCAT PDO Receive3 : slrealtimeethercatlib/EtherCAT PDO Receive  Priority=2  sig_name=Box 1 (PIC32 EtherCAT Slave01).INPUTS process data mapping.IMU1_X  sig_offset=952  sig_type=single  type_size=32  sig_dim=1  device_id=0  sample_time=0.001000
  EtherCAT PDO Receive4 : slrealtimeethercatlib/EtherCAT PDO Receive  Priority=2  sig_name=Box 1 (PIC32 EtherCAT Slave01).INPUTS process data mapping.IMU1_Y  sig_offset=984  sig_type=single  type_size=32  sig_dim=1  device_id=0  sample_time=0.001000
  EtherCAT PDO Receive5 : slrealtimeethercatlib/EtherCAT PDO Receive  Priority=2  sig_name=Box 1 (PIC32 EtherCAT Slave01).INPUTS process data mapping.IMU1_Z  sig_offset=1016  sig_type=single  type_size=32  sig_dim=1  device_id=0  sample_time=0.001000
  EtherCAT PDO Receive6 : slrealtimeethercatlib/EtherCAT PDO Receive  Priority=2  sig_name=Box 1 (PIC32 EtherCAT Slave01).INPUTS process data mapping.IMU2_X  sig_offset=1048  sig_type=single  type_size=32  sig_dim=1  device_id=0  sample_time=0.001000
  EtherCAT PDO Receive7 : slrealtimeethercatlib/EtherCAT PDO Receive  Priority=2  sig_name=Box 1 (PIC32 EtherCAT Slave01).INPUTS process data mapping.FORCE3  sig_offset=760  sig_type=single  type_size=32  sig_dim=1  device_id=0  sample_time=0.001000
  Out1 : Outport
  Out2 : Outport  Port=2
  Out3 : Outport  Port=3
  Out4 : Outport  Port=4
  Out5 : Outport  Port=5
  Out6 : Outport  Port=6
  Out7 : Outport  Port=7
  wires:
  EtherCAT PDO Receive1/1 -> Out1/1
  EtherCAT PDO Receive2/1 -> Out2/1
  EtherCAT PDO Receive3/1 -> Out3/1
  EtherCAT PDO Receive4/1 -> Out4/1
  EtherCAT PDO Receive5/1 -> Out5/1
  EtherCAT PDO Receive6/1 -> Out6/1
  EtherCAT PDO Receive7/1 -> Out7/1

== system TestStructure/Bus/Subsystem6/Enabled Subsystem/Subsystem8 ==
  EtherCAT PDO Receive1 : slrealtimeethercatlib/EtherCAT PDO Receive  Priority=2  sig_name=Box 1 (PIC32 EtherCAT Slave01).INPUTS process data mapping.FORCE1  sig_offset=696  sig_type=single  type_size=32  sig_dim=1  device_id=0  sample_time=0.001000
  EtherCAT PDO Receive2 : slrealtimeethercatlib/EtherCAT PDO Receive  Priority=2  sig_name=Box 1 (PIC32 EtherCAT Slave01).INPUTS process data mapping.FORCE2  sig_offset=728  sig_type=single  type_size=32  sig_dim=1  device_id=0  sample_time=0.001000
  EtherCAT PDO Receive3 : slrealtimeethercatlib/EtherCAT PDO Receive  Priority=2  sig_name=Box 1 (PIC32 EtherCAT Slave01).INPUTS process data mapping.IMU1_X  sig_offset=952  sig_type=single  type_size=32  sig_dim=1  device_id=0  sample_time=0.001000
  EtherCAT PDO Receive4 : slrealtimeethercatlib/EtherCAT PDO Receive  Priority=2  sig_name=Box 1 (PIC32 EtherCAT Slave01).INPUTS process data mapping.IMU1_Y  sig_offset=984  sig_type=single  type_size=32  sig_dim=1  device_id=0  sample_time=0.001000
  EtherCAT PDO Receive5 : slrealtimeethercatlib/EtherCAT PDO Receive  Priority=2  sig_name=Box 1 (PIC32 EtherCAT Slave01).INPUTS process data mapping.IMU1_Z  sig_offset=1016  sig_type=single  type_size=32  sig_dim=1  device_id=0  sample_time=0.001000
  EtherCAT PDO Receive6 : slrealtimeethercatlib/EtherCAT PDO Receive  Priority=2  sig_name=Box 1 (PIC32 EtherCAT Slave01).INPUTS process data mapping.IMU2_X  sig_offset=1048  sig_type=single  type_size=32  sig_dim=1  device_id=0  sample_time=0.001000
  EtherCAT PDO Receive7 : slrealtimeethercatlib/EtherCAT PDO Receive  Priority=2  sig_name=Box 1 (PIC32 EtherCAT Slave01).INPUTS process data mapping.FORCE3  sig_offset=760  sig_type=single  type_size=32  sig_dim=1  device_id=0  sample_time=0.001000
  Out1 : Outport
  Out2 : Outport  Port=2
  Out3 : Outport  Port=3
  Out4 : Outport  Port=4
  Out5 : Outport  Port=5
  Out6 : Outport  Port=6
  Out7 : Outport  Port=7
  wires:
  EtherCAT PDO Receive1/1 -> Out1/1
  EtherCAT PDO Receive2/1 -> Out2/1
  EtherCAT PDO Receive3/1 -> Out3/1
  EtherCAT PDO Receive4/1 -> Out4/1
  EtherCAT PDO Receive5/1 -> Out5/1
  EtherCAT PDO Receive6/1 -> Out6/1
  EtherCAT PDO Receive7/1 -> Out7/1

== system TestStructure/Bus/Subsystem6/Enabled Subsystem/Subsystem9 ==
  EtherCAT PDO Receive1 : slrealtimeethercatlib/EtherCAT PDO Receive  Priority=2  sig_name=Box 1 (PIC32 EtherCAT Slave01).INPUTS process data mapping.FORCE1  sig_offset=696  sig_type=single  type_size=32  sig_dim=1  device_id=0  sample_time=0.001000
  EtherCAT PDO Receive2 : slrealtimeethercatlib/EtherCAT PDO Receive  Priority=2  sig_name=Box 1 (PIC32 EtherCAT Slave01).INPUTS process data mapping.FORCE2  sig_offset=728  sig_type=single  type_size=32  sig_dim=1  device_id=0  sample_time=0.001000
  EtherCAT PDO Receive3 : slrealtimeethercatlib/EtherCAT PDO Receive  Priority=2  sig_name=Box 1 (PIC32 EtherCAT Slave01).INPUTS process data mapping.IMU1_X  sig_offset=952  sig_type=single  type_size=32  sig_dim=1  device_id=0  sample_time=0.001000
  EtherCAT PDO Receive4 : slrealtimeethercatlib/EtherCAT PDO Receive  Priority=2  sig_name=Box 1 (PIC32 EtherCAT Slave01).INPUTS process data mapping.IMU1_Y  sig_offset=984  sig_type=single  type_size=32  sig_dim=1  device_id=0  sample_time=0.001000
  EtherCAT PDO Receive5 : slrealtimeethercatlib/EtherCAT PDO Receive  Priority=2  sig_name=Box 1 (PIC32 EtherCAT Slave01).INPUTS process data mapping.IMU1_Z  sig_offset=1016  sig_type=single  type_size=32  sig_dim=1  device_id=0  sample_time=0.001000
  EtherCAT PDO Receive6 : slrealtimeethercatlib/EtherCAT PDO Receive  Priority=2  sig_name=Box 1 (PIC32 EtherCAT Slave01).INPUTS process data mapping.IMU2_X  sig_offset=1048  sig_type=single  type_size=32  sig_dim=1  device_id=0  sample_time=0.001000
  EtherCAT PDO Receive7 : slrealtimeethercatlib/EtherCAT PDO Receive  Priority=2  sig_name=Box 1 (PIC32 EtherCAT Slave01).INPUTS process data mapping.FORCE3  sig_offset=760  sig_type=single  type_size=32  sig_dim=1  device_id=0  sample_time=0.001000
  Out1 : Outport
  Out2 : Outport  Port=2
  Out3 : Outport  Port=3
  Out4 : Outport  Port=4
  Out5 : Outport  Port=5
  Out6 : Outport  Port=6
  Out7 : Outport  Port=7
  wires:
  EtherCAT PDO Receive1/1 -> Out1/1
  EtherCAT PDO Receive2/1 -> Out2/1
  EtherCAT PDO Receive3/1 -> Out3/1
  EtherCAT PDO Receive4/1 -> Out4/1
  EtherCAT PDO Receive5/1 -> Out5/1
  EtherCAT PDO Receive6/1 -> Out6/1
  EtherCAT PDO Receive7/1 -> Out7/1

== system TestStructure/Bus/Subsystem6/Subsystem/Subsystem ==
  In1 : Inport
  In2 : Inport  Port=2
  In3 : Inport  Port=3
  In4 : Inport  Port=4
  EtherCAT PDO Receive1 : slrealtimeethercatlib/EtherCAT PDO Receive  Priority=2  sig_name=Box 1 (PIC32 EtherCAT Slave01).INPUTS process data mapping.FORCE1  sig_offset=696  sig_type=single  type_size=32  sig_dim=1  device_id=0  sample_time=0.001
  EtherCAT PDO Receive2 : slrealtimeethercatlib/EtherCAT PDO Receive  Priority=2  sig_name=Box 1 (PIC32 EtherCAT Slave01).INPUTS process data mapping.FORCE2  sig_offset=728  sig_type=single  type_size=32  sig_dim=1  device_id=0  sample_time=0.001000
  EtherCAT PDO Receive3 : slrealtimeethercatlib/EtherCAT PDO Receive  Priority=2  sig_name=Box 1 (PIC32 EtherCAT Slave01).INPUTS process data mapping.IMU1_X  sig_offset=952  sig_type=single  type_size=32  sig_dim=1  device_id=0  sample_time=0.001000
  EtherCAT PDO Receive4 : slrealtimeethercatlib/EtherCAT PDO Receive  Priority=2  sig_name=Box 1 (PIC32 EtherCAT Slave01).INPUTS process data mapping.IMU1_Y  sig_offset=984  sig_type=single  type_size=32  sig_dim=1  device_id=0  sample_time=0.001000
  EtherCAT PDO Receive5 : slrealtimeethercatlib/EtherCAT PDO Receive  Priority=2  sig_name=Box 1 (PIC32 EtherCAT Slave01).INPUTS process data mapping.IMU1_Z  sig_offset=1016  sig_type=single  type_size=32  sig_dim=1  device_id=0  sample_time=0.001000
  EtherCAT PDO Receive6 : slrealtimeethercatlib/EtherCAT PDO Receive  Priority=2  sig_name=Box 1 (PIC32 EtherCAT Slave01).INPUTS process data mapping.IMU2_X  sig_offset=1048  sig_type=single  type_size=32  sig_dim=1  device_id=0  sample_time=0.001000
  EtherCAT PDO Receive7 : slrealtimeethercatlib/EtherCAT PDO Receive  Priority=2  sig_name=Box 1 (PIC32 EtherCAT Slave01).INPUTS process data mapping.FORCE3  sig_offset=760  sig_type=single  type_size=32  sig_dim=1  device_id=0  sample_time=0.001000
  EtherCAT PDO Receive8 : slrealtimeethercatlib/EtherCAT PDO Receive  Priority=2  sig_name=Box 1 (PIC32 EtherCAT Slave01).INPUTS process data mapping.FORCE3  sig_offset=760  sig_type=single  type_size=32  sig_dim=1  device_id=0  sample_time=0.001000
  EtherCAT PDO Receive9 : slrealtimeethercatlib/EtherCAT PDO Receive  Priority=2  sig_name=Box 1 (PIC32 EtherCAT Slave01).INPUTS process data mapping.FORCE3  sig_offset=760  sig_type=single  type_size=32  sig_dim=1  device_id=0  sample_time=0.001000
  EtherCAT PDO Transmit{,1..3} (4 alike) : slrealtimeethercatlib/EtherCAT PDO Transmit  Priority=5  sig_name=Drive 2 (Elmo Drive ).Outputs.Target Torque  sig_offset=12496  sig_type=int16  type_size=16  sig_dim=1  device_id=0  sample_time=0.001000
  Out1 : Outport
  Out2 : Outport  Port=2
  Out3 : Outport  Port=3
  Out4 : Outport  Port=4
  Out5 : Outport  Port=5
  Out6 : Outport  Port=6
  Out7 : Outport  Port=7
  Out8 : Outport  Port=8
  Out9 : Outport  Port=9
  wires:
  EtherCAT PDO Receive1/1 -> Out1/1
  EtherCAT PDO Receive2/1 -> Out2/1
  EtherCAT PDO Receive3/1 -> Out3/1
  EtherCAT PDO Receive4/1 -> Out4/1
  EtherCAT PDO Receive5/1 -> Out5/1
  EtherCAT PDO Receive6/1 -> Out6/1
  EtherCAT PDO Receive7/1 -> Out7/1
  EtherCAT PDO Receive8/1 -> Out8/1
  EtherCAT PDO Receive9/1 -> Out9/1
  In1/1 -> EtherCAT PDO Transmit/1
  In2/1 -> EtherCAT PDO Transmit1/1
  In4/1 -> EtherCAT PDO Transmit2/1
  In3/1 -> EtherCAT PDO Transmit3/1

== system TestStructure/Bus/Subsystem6/Subsystem/Subsystem1 ==
  In1 : Inport
  EtherCAT PDO Receive1 : slrealtimeethercatlib/EtherCAT PDO Receive  Priority=2  sig_name=Drive 3 (Elmo Drive ).Inputs.Position actual value  sig_offset=1432  sig_type=int32  type_size=32  sig_dim=1  device_id=0  sample_time=0.001000
  EtherCAT PDO Receive2 : slrealtimeethercatlib/EtherCAT PDO Receive  Priority=2  sig_name=Drive 3 (Elmo Drive ).Inputs_1.Velocity actual value  sig_offset=1512  sig_type=int32  type_size=32  sig_dim=1  device_id=0  sample_time=0.001000
  EtherCAT PDO Receive3 : slrealtimeethercatlib/EtherCAT PDO Receive  Priority=2  sig_name=Drive 3 (Elmo Drive ).Inputs.Torque actual value  sig_offset=1464  sig_type=int16  type_size=16  sig_dim=1  device_id=0  sample_time=0.001000
  EtherCAT PDO Receive4 : slrealtimeethercatlib/EtherCAT PDO Receive  Priority=2  sig_name=Drive 3 (Elmo Drive ).Inputs_2.DC link circuit voltage  sig_offset=1544  sig_type=uint32  type_size=32  sig_dim=1  device_id=0  sample_time=0.001000
  EtherCAT PDO Receive5 : slrealtimeethercatlib/EtherCAT PDO Receive  Priority=2  sig_name=Drive 3 (Elmo Drive ).Inputs.Mode of operation display  sig_offset=1496  sig_type=int8  type_size=8  sig_dim=1  device_id=0  sample_time=0.001000
  EtherCAT PDO Transmit : slrealtimeethercatlib/EtherCAT PDO Transmit  Priority=5  Commented=on  sig_name=Drive 2 (Elmo Drive ).Outputs.Target Torque  sig_offset=12496  sig_type=int16  type_size=16  sig_dim=1  device_id=0  sample_time=0.001000
  Out1 : Outport
  Out2 : Outport  Port=2
  Out3 : Outport  Port=3
  Out4 : Outport  Port=4
  Out5 : Outport  Port=5
  wires:
  In1/1 -> EtherCAT PDO Transmit/1
  EtherCAT PDO Receive5/1 -> Out5/1
  EtherCAT PDO Receive4/1 -> Out4/1
  EtherCAT PDO Receive3/1 -> Out3/1
  EtherCAT PDO Receive2/1 -> Out2/1
  EtherCAT PDO Receive1/1 -> Out1/1

== system TestStructure/Bus/Subsystem6/Subsystem/Subsystem10 ==
  EtherCAT PDO Receive1 : slrealtimeethercatlib/EtherCAT PDO Receive  Priority=2  sig_name=Box 1 (PIC32 EtherCAT Slave01).INPUTS process data mapping.FORCE1  sig_offset=696  sig_type=single  type_size=32  sig_dim=1  device_id=0  sample_time=0.001000
  EtherCAT PDO Receive2 : slrealtimeethercatlib/EtherCAT PDO Receive  Priority=2  sig_name=Box 1 (PIC32 EtherCAT Slave01).INPUTS process data mapping.FORCE2  sig_offset=728  sig_type=single  type_size=32  sig_dim=1  device_id=0  sample_time=0.001000
  EtherCAT PDO Receive3 : slrealtimeethercatlib/EtherCAT PDO Receive  Priority=2  sig_name=Box 1 (PIC32 EtherCAT Slave01).INPUTS process data mapping.IMU1_X  sig_offset=952  sig_type=single  type_size=32  sig_dim=1  device_id=0  sample_time=0.001000
  EtherCAT PDO Receive4 : slrealtimeethercatlib/EtherCAT PDO Receive  Priority=2  sig_name=Box 1 (PIC32 EtherCAT Slave01).INPUTS process data mapping.IMU1_Y  sig_offset=984  sig_type=single  type_size=32  sig_dim=1  device_id=0  sample_time=0.001000
  EtherCAT PDO Receive5 : slrealtimeethercatlib/EtherCAT PDO Receive  Priority=2  sig_name=Box 1 (PIC32 EtherCAT Slave01).INPUTS process data mapping.IMU1_Z  sig_offset=1016  sig_type=single  type_size=32  sig_dim=1  device_id=0  sample_time=0.001000
  EtherCAT PDO Receive6 : slrealtimeethercatlib/EtherCAT PDO Receive  Priority=2  sig_name=Box 1 (PIC32 EtherCAT Slave01).INPUTS process data mapping.IMU2_X  sig_offset=1048  sig_type=single  type_size=32  sig_dim=1  device_id=0  sample_time=0.001000
  EtherCAT PDO Receive7 : slrealtimeethercatlib/EtherCAT PDO Receive  Priority=2  sig_name=Box 1 (PIC32 EtherCAT Slave01).INPUTS process data mapping.FORCE3  sig_offset=760  sig_type=single  type_size=32  sig_dim=1  device_id=0  sample_time=0.001000
  Out1 : Outport
  Out2 : Outport  Port=2
  Out3 : Outport  Port=3
  Out4 : Outport  Port=4
  Out5 : Outport  Port=5
  Out6 : Outport  Port=6
  Out7 : Outport  Port=7
  wires:
  EtherCAT PDO Receive1/1 -> Out1/1
  EtherCAT PDO Receive2/1 -> Out2/1
  EtherCAT PDO Receive3/1 -> Out3/1
  EtherCAT PDO Receive4/1 -> Out4/1
  EtherCAT PDO Receive5/1 -> Out5/1
  EtherCAT PDO Receive6/1 -> Out6/1
  EtherCAT PDO Receive7/1 -> Out7/1
